simulink subsystem "Nitrous_Tank_Custom_h"  (R2020b)
settings: Solver=VariableStepAuto  StartTime=0.0  StopTime=10.0  RelTol=1e-3
model mask{nitrousLiqConCrossSection=3.8485e-05, nitrousVapConCrossSection=2e-5, nitrousTankVol=0.0141, initialTankPressure=60e5, initialLiqMassFraction=0.7, totalHeatTransferSurfaceArea=6, heatTranferWallToLiq=0, heatTranferWallToVap=0}
  mask prompts: nitrousLiqConCrossSection "Liquid port cross section in m^2"; nitrousVapConCrossSection "Vapour port cross section in m^2"; nitrousTankVol "Tank Volume in m^3"; initialTankPressure "Tank start pressure in Pa"; initialLiqMassFraction "Fraction of the nitrous in the tank which starts out liquid (By mass)"; totalHeatTransferSurfaceArea "Total heat transfer surface area (inner wall) m^2"; heatTranferWallToLiq "Heat transfer coefficient wall to liquid"; heatTranferWallToVap "Heat transfer coefficient wall to vapour"
libraries: nesl_utility x6, fl_lib x2, SimscapeCustomBlocks_lib x2
settings Model: Creator=luc  LastModifiedBy=luc

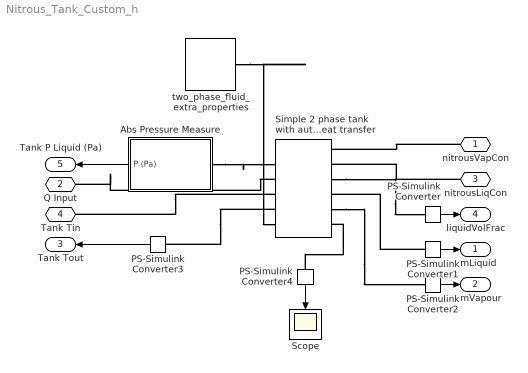
== system Nitrous_Tank_Custom_h ==
  Abs Pressure Measure : Subsystem
  PS-Simulink Converter{,1..4} (5 alike) : nesl_utility/PS-Simulink Converter  PhysicalDomain=network_engine_domain  SubClassName=ps_output  LeftPortType=input  RightPortType=output  PseudoPeriodic=off  Frequencies=[]  Unit=inherit  AffineConversion=off
  Scope : Scope
  Simple 2 phase tank with automatic heat transfer : SimscapeCustomBlocks_lib/Simple 2 phase tank with automatic heat transfer  areaL=nitrousLiqConCrossSection m^2  areaV=nitrousVapConCrossSection m^2  tank_volume=nitrousTankVol m^3  heat_surface_area=totalHeatTransferSurfaceArea m^2  wall_thickness=0.002 m  g=9.8 m/s^2  p_init=initialTankPressure Pa  liq_vol_frac_init=initialLiqMassFraction
      settings: InternalSimscapePortConfiguration="{\"Bottom\":[{\"id\":\"beta\",\"label\":\"beta\",\"type\":\"output\"}],\"Left\":[{\"id\":\"AV\",\"label\":\"AV\",\"type\":\"foundation.two_phase_fluid.two_phase_fluid\"},{\"id\":\"AL\",\"label\":\"AL\",\"type\":\"foundation.two_phase_fluid.two_phase_fluid\"},{\"id\":\"H\",\"label\":\"H\",\"type\":\"foundation.thermal.thermal\"},{\"id\":\"T_external\",\"label\":\"Tin\",\"type\":\"input\"},{\"id\":\"T\",\"label\":\"Tout\",\"type\":\"output\"}],\"Right\":[{\"id\":\"BV\",\"label\":\"BV\",\"type\":\"foundation.two_phase_fluid.two_phase_fluid\"},{\"id\":\"BL\",\"label\":\"BL\",\"type\":\"foundation.two_phase_fluid.two_phase_fluid\"},{\"id\":\"L\",\"label\":\"L\",\"type\":\"output\"},{\"id\":\"ML\",\"label\":\"ML\",\"type\":\"output\"},{\"id\":\"MV\",\"label\":\"MV\",\"type\":\"output\"}],\"Top\":[{\"id\":\"Props\",\"label\":\"Props\",\"type\":\"SimscapeCustomBlocks.customFluidDomain.extra_two_phase_fluid_props\"}]}"
  two_phase_fluid_extra_properties : SimscapeCustomBlocks_lib/two_phase_fluid_extra_properties  unorm_liq=Sim.extraNitrousPropsTable.liquid.unorm  unorm_vap=Sim.extraNitrousPropsTable.vapor.unorm  p_TLU=Sim.extraNitrousPropsTable.p MPa  Cp_liq=Sim.extraNitrousPropsTable.liquid.cp J/kg/K  Cp_vap=Sim.extraNitrousPropsTable.vapor.cp J/kg/K  Cv_liq=Sim.extraNitrousPropsTable.liquid.cv J/kg/K  Cv_vap=Sim.extraNitrousPropsTable.vapor.cv J/kg/K  PVap_liq=Sim.extraNitrousPropsTable.liquid.pvap MPa  PVap_vap=Sim.extraNitrousPropsTable.vapor.pvap MPa  beta_vap=Sim.extraNitrousPropsTable.vapor.beta 1/K  beta_liq=Sim.extraNitrousPropsTable.liquid.beta 1/K
      settings: InternalSimscapePortConfiguration="{\"Bottom\":[],\"Left\":[],\"Right\":[{\"id\":\"A\",\"label\":\"A\",\"type\":\"SimscapeCustomBlocks.customFluidDomain.extra_two_phase_fluid_props\"}],\"Top\":[]}"
  nitrousVapCon : PMIOPort  Side=Left
  Q Input : PMIOPort  Port=2  Side=Left
  nitrousLiqCon : PMIOPort  Port=3  Side=Right
  Tank Tin : PMIOPort  Port=4  Side=Left
  mLiquid : Outport
  mVapour : Outport  Port=2
  Tank Tout : Outport  Port=3
  liquidVolFrac : Outport  Port=4
  Tank P Liquid (Pa) : Outport  Port=5
  wires:
  Abs Pressure Measure/1(P (Pa)) -> Tank P Liquid (Pa)/1
  PS-Simulink Converter/1 -> liquidVolFrac/1
  PS-Simulink Converter1/1 -> mLiquid/1
  PS-Simulink Converter2/1 -> mVapour/1
  PS-Simulink Converter3/1 -> Tank Tout/1
  PS-Simulink Converter4/1 -> Scope/1
  connections:
  Abs Pressure Measure/LConn1 -- Simple 2 phase tank with automatic heat transfer/LConn2
  nitrousLiqCon/RConn1 -- Simple 2 phase tank with automatic heat transfer/RConn2
  Simple 2 phase tank with automatic heat transfer/LConn3 -- Q Input/RConn1
  nitrousVapCon/RConn1 -- Simple 2 phase tank with automatic heat transfer/RConn1
  Simple 2 phase tank with automatic heat transfer/RConn5 -- PS-Simulink Converter2/LConn1
  PS-Simulink Converter1/LConn1 -- Simple 2 phase tank with automatic heat transfer/RConn4
  Simple 2 phase tank with automatic heat transfer/RConn3 -- PS-Simulink Converter/LConn1
  two_phase_fluid_extra_properties/RConn1 -- Simple 2 phase tank with automatic heat transfer/LConn6
  Simple 2 phase tank with automatic heat transfer/LConn5 -- PS-Simulink Converter3/LConn1
  PS-Simulink Converter4/LConn1 -- Simple 2 phase tank with automatic heat transfer/RConn6
  Simple 2 phase tank with automatic heat transfer/LConn4 -- Tank Tin/RConn1

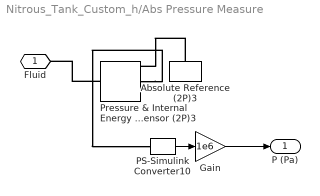
== system Nitrous_Tank_Custom_h/Abs Pressure Measure ==
  Absolute Reference (2P)3 : fl_lib/Two-Phase Fluid/Elements/Absolute Reference (2P)
      settings: SourceProductBaseCode=SS
  Gain : Gain  Gain=1e6
  PS-Simulink Converter10 : nesl_utility/PS-Simulink Converter  PhysicalDomain=network_engine_domain  SubClassName=ps_output  LeftPortType=input  RightPortType=output  PseudoPeriodic=off  Frequencies=[]  Unit=inherit  AffineConversion=off
  Pressure & Internal Energy Sensor (2P)3 : fl_lib/Two-Phase Fluid/Sensors/Pressure & Internal Energy Sensor (2P)
      settings: SourceProductBaseCode=SS  InternalSimscapePortConfiguration="{\"Bottom\":[],\"Left\":[{\"id\":\"A\",\"label\":\"A\",\"type\":\"foundation.two_phase_fluid.two_phase_fluid\"}],\"Right\":[{\"id\":\"B\",\"label\":\"B\",\"type\":\"foundation.two_phase_fluid.two_phase_fluid\"},{\"id\":\"P\",\"label\":\"P\",\"type\":\"output\"},{\"id\":\"U\",\"label\":\"U\",\"type\":\"output\"}],\"Top\":[]}"
  Fluid : PMIOPort  Side=Left
  P (Pa) : Outport
  wires:
  Gain/1 -> P (Pa)/1
  PS-Simulink Converter10/1 -> Gain/1
  connections:
  Pressure & Internal Energy Sensor (2P)3/LConn1 -- Fluid/RConn1
  Pressure & Internal Energy Sensor (2P)3/RConn2 -- PS-Simulink Converter10/LConn1
  Absolute Reference (2P)3/LConn1 -- Pressure & Internal Energy Sensor (2P)3/RConn1
